simulink model "Inverted_Pendulum"  (R2018a)
settings: Solver=ode45  StartTime=0.0  StopTime=20  RelTol=1e-3
undefined symbols (not defined in the file or in its folder): Inv
libraries: vrlib x4, simulink x1, realtime_pacer_lib x1, sharedtransform x1
settings Model: Creator=Jarvis  LastModifiedBy=Jarvis
settings SolverCC: AlgebraicLoopSolver=LineSearch
settings DebuggingCC: AlgebraicLoopMsg=none

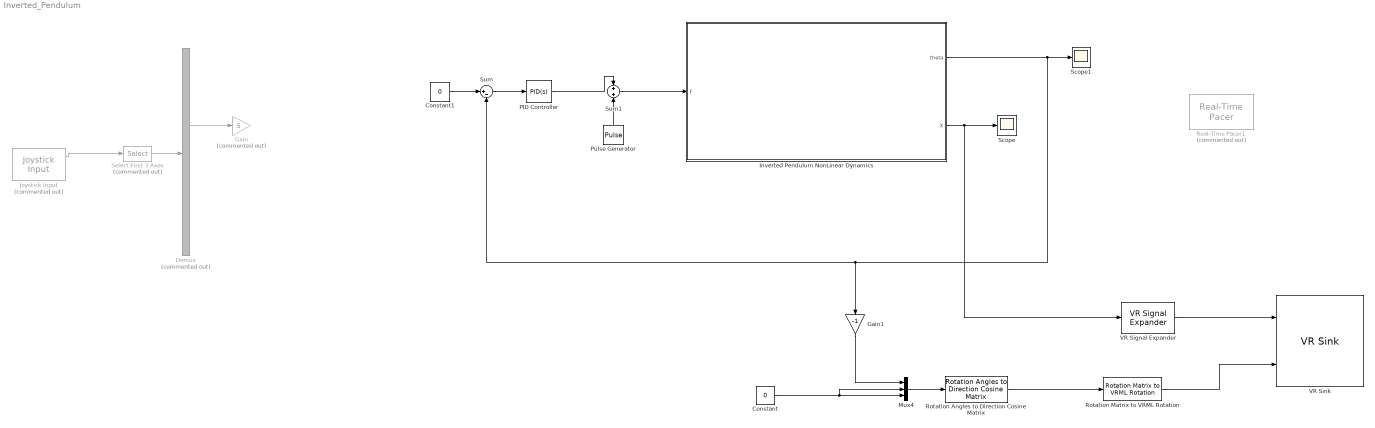
== system Inverted_Pendulum ==
  Constant : Constant  Value=0
  Constant1 : Constant  Value=0
  Demux : Demux  Commented=on
  Gain : Gain  Commented=on  Gain=5
  Gain1 : Gain  Gain=-1
  Inverted Pendulum NonLinear Dynamics : Subsystem
  Joystick Input : vrlib/Joystick Input  Commented=on  joyid=1  adjustports=on  forcefeed=off
      settings: SourceProductBaseCode=VR
  Mux4 : Mux  Inputs=3
  PID Controller : simulink/Continuous/PID Controller  Controller=PID  TimeDomain=Continuous-time  SampleTime=-1  IntegratorMethod=Forward Euler  FilterMethod=Forward Euler  Form=Parallel  UseFilter=on  ControllerParametersSource=internal  P=22.76603508324  I=38.0034206492837  D=3.3509902387091  N=2377.77482545523  InitialConditionSource=internal  InitialConditionForIntegrator=0  InitialConditionForFilter=0  ExternalReset=none  LimitOutput=off  UpperSaturationLimit=inf  LowerSaturationLimit=-inf  LinearizeAsGain=on  AntiWindupMode=none  Kb=1  TrackingMode=off  Kt=1  PParamMin=[]  PParamMax=[]  IParamMin=[]  IParamMax=[]  DParamMin=[]  DParamMax=[]  NParamMin=[]  NParamMax=[]  KbParamMin=[]  KbParamMax=[]  KtParamMin=[]  KtParamMax=[]  POutMin=[]  POutMax=[]  IOutMin=[]  IOutMax=[]  DOutMin=[]  DOutMax=[]  NOutMin=[]  NOutMax=[]  KbOutMin=[]  KbOutMax=[]  KtOutMin=[]  KtOutMax=[]  IntegratorOutMin=[]  IntegratorOutMax=[]  FilterOutMin=[]  FilterOutMax=[]  SumOutMin=[]  SumOutMax=[]  SumI1OutMin=[]  SumI1OutMax=[]  SumI2OutMin=[]  SumI2OutMax=[]  SumI3OutMin=[]  SumI3OutMax=[]  SumDOutMin=[]  SumDOutMax=[]  SaturationOutMin=[]  SaturationOutMax=[]  IntegratorContinuousStateAttributes=''  IntegratorStateMustResolveToSignalObject=off  IntegratorRTWStateStorageClass=Auto  FilterContinuousStateAttributes=''  FilterStateMustResolveToSignalObject=off  FilterRTWStateStorageClass=Auto  DifferentiatorICPrevScaledInput=0  DifferentiatorOutMin=[]  DifferentiatorOutMax=[]  FilterDiffOutCoefMin=[]  FilterDiffOutCoefMax=[]  SumDenOutMin=[]  SumDenOutMax=[]  SumNumOutMin=[]  SumNumOutMax=[]  ReciprocalOutMin=[]  ReciprocalOutMax=[]  DivideOutMin=[]  DivideOutMax=[]  TunerSelectOption=Transfer Function Based (PID Tuner App)
  Pulse Generator : DiscretePulseGenerator  PulseType=Time based  Amplitude=500  Period=1000  PulseWidth=0.001  PhaseDelay=10
  Real-Time Pacer1 : realtime_pacer_lib/Real-Time Pacer  Commented=on  simTimePerRealTime=1
  Rotation Angles to Direction Cosine Matrix : sharedtransform/Rotation Angles to Direction Cosine Matrix  rotationOrder=ZYX  aMode=aMode
      settings: SourceProductBaseCode=AE
  Rotation Matrix to VRML Rotation : vrlib/Utilities/Rotation Matrix to VRML Rotation  maxzero=1e-12
      settings: SourceProductName=Simulink 3D Animation  SourceProductBaseCode=VR
  Scope : Scope
  Scope1 : Scope
  Select First 3 Axes : Selector  Commented=on  InputPortWidth=5  IndexOptions=Index vector (dialog)  Indices=[1 2 3 4]  OutputSizes=1
      settings: AttributesFormatString=(Joystick - dependent)
  Sum : Sum  Inputs=|+-
  Sum1 : Sum
  VR Signal Expander : vrlib/VR Signal Expander  outwidth=3  outidx=[1]
      settings: SourceProductName=Simulink 3D Animation  SourceProductBaseCode=VR
  VR Sink : vrlib/VR Sink  InstantiateOnLoad=on  SampleTime=0.01  ViewEnable=on  RemoteChange=off  RemoteView=off  FieldsWritten=Cart.translation.3.1.1.double#Pendulum.rotation.4.1.1.double  WorldFileName=Inverted_Pendulum.wrl  AutoView=off  VideoDimensions=[]  AllowVariableSize=off
      settings: SourceProductBaseCode=VR
  wires:
  Sum/1 -> PID Controller/1
  Inverted Pendulum NonLinear Dynamics/1(theta) -> Sum/2, Gain1/1, Scope1/1
  Inverted Pendulum NonLinear Dynamics/2(X) -> VR Signal Expander/1, Scope/1
  VR Signal Expander/1 -> VR Sink/1
  Mux4/1 -> Rotation Angles to Direction Cosine Matrix/1
  Rotation Angles to Direction Cosine Matrix/1 -> Rotation Matrix to VRML Rotation/1
  Constant/1 -> Mux4/3, Mux4/2
  Rotation Matrix to VRML Rotation/1 -> VR Sink/2
  Select First 3 Axes/1 -> Demux/1
  Demux/2 -> Gain/1
  Joystick Input/1 -> Select First 3 Axes/1
  Gain1/1 -> Mux4/1
  PID Controller/1 -> Sum1/1
  Sum1/1 -> Inverted Pendulum NonLinear Dynamics/1(F)
  Constant1/1 -> Sum/1
  Pulse Generator/1 -> Sum1/2

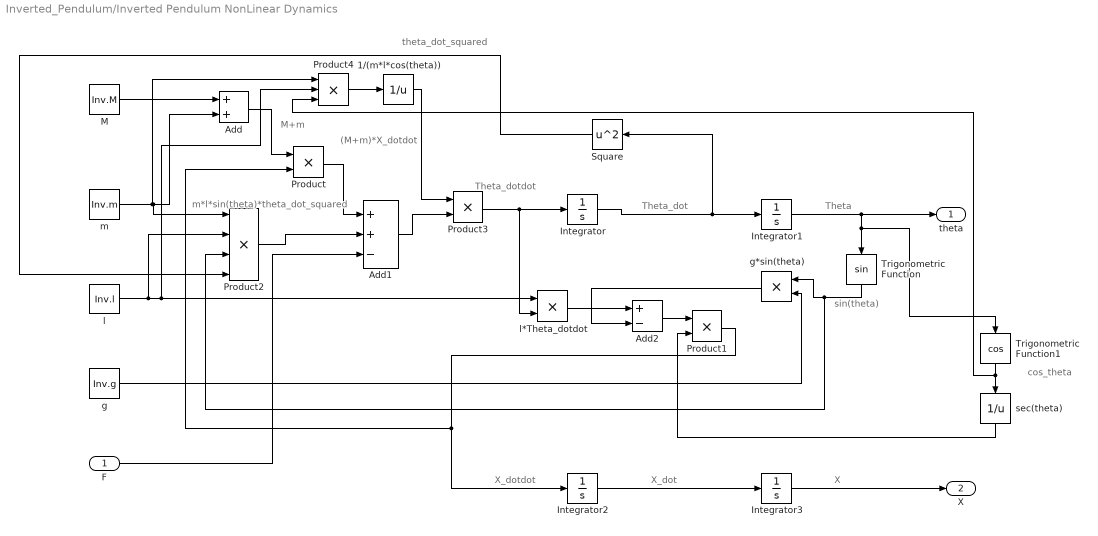
== system Inverted_Pendulum/Inverted Pendulum NonLinear Dynamics ==
  note: m*l*sin(theta)*theta_dot_squared
  note: theta_dot_squared
  note: sin(theta)
  note: cos_theta
  note: X_dotdot
  note: Theta_dotdot
  note: M+m
  note: Theta_dot
  note: Theta
  note: X
  note: X_dot
  note: (M+m)*X_dotdot
  F : Inport
  1/(m*l*cos(theta)) : Math  Operator=reciprocal  SaturateOnIntegerOverflow=on
  Add : Sum
  Add1 : Sum  Inputs=++-
  Add2 : Sum  Inputs=+-
  Integrator{,1..3} (4 alike) : Integrator
  M : Constant  Value=Inv.M
  Product : Product
  Product1 : Product
  Product2 : Product  Inputs=4
  Product3 : Product
  Product4 : Product  Inputs=3
  Square : Math  Operator=square  SaturateOnIntegerOverflow=on
  Trigonometric Function : Trigonometry
  Trigonometric Function1 : Trigonometry  Operator=cos
  g : Constant  Value=Inv.g
  g*sin(theta) : Product
  l : Constant  Value=Inv.l
  l*Theta_dotdot : Product
  m : Constant  Value=Inv.m
  "sec(theta)    " : Math  Operator=reciprocal  SaturateOnIntegerOverflow=on
  theta : Outport
  X : Outport  Port=2
  wires:
  Integrator/1 -> Square/1, Integrator1/1
  Integrator2/1 -> Integrator3/1
  M/1 -> Add/1
  m/1 -> Product4/1, Product2/1, Add/2
  Add/1 -> Product/1
  Product/1 -> Add1/1
  Add1/1 -> Product3/2
  Product3/1 -> l*Theta_dotdot/2, Integrator/1
  Integrator1/1 -> Trigonometric Function1/1, Trigonometric Function/1, theta/1
  Integrator3/1 -> X/1
  l/1 -> Product4/2, l*Theta_dotdot/1, Product2/2
  l*Theta_dotdot/1 -> Add2/1
  g/1 -> g*sin(theta)/2
  g*sin(theta)/1 -> Add2/2
  Product1/1 -> Product/2, Integrator2/1
  Trigonometric Function/1 -> Product2/3, g*sin(theta)/1
  Trigonometric Function1/1 -> Product4/3, "sec(theta)    "/1
  Add2/1 -> Product1/1
  "sec(theta)    "/1 -> Product1/2
  Square/1 -> Product2/4
  F/1 -> Add1/3
  Product2/1 -> Add1/2
  Product4/1 -> 1/(m*l*cos(theta))/1
  1/(m*l*cos(theta))/1 -> Product3/1
